simulink model "Example_InterpretedFunction"  (R2024a)
settings: Solver=VariableStepAuto  StartTime=0.0  StopTime=10.0  RelTol=1e-3
values from neighbouring files (symbols this model uses):
  x = acosd(y)    [MATLAB_Cheat_Sheet_Practice.m]
  y = pi    (= 3.14159265359)    [MATLAB_Cheat_Sheet_Practice.m]
undefined symbols (not defined in the file or in its folder): Hello___Matlab
settings Model: Creator=AbdelrahmanMourad  LastModifiedBy=AbdelrahmanMourad

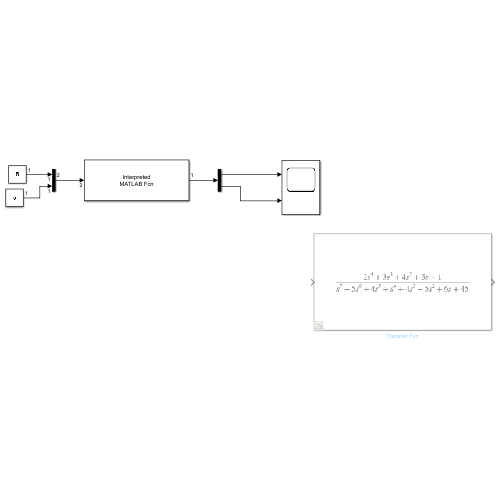
[thumbnail: Simulink's stored preview of the top-level diagram]
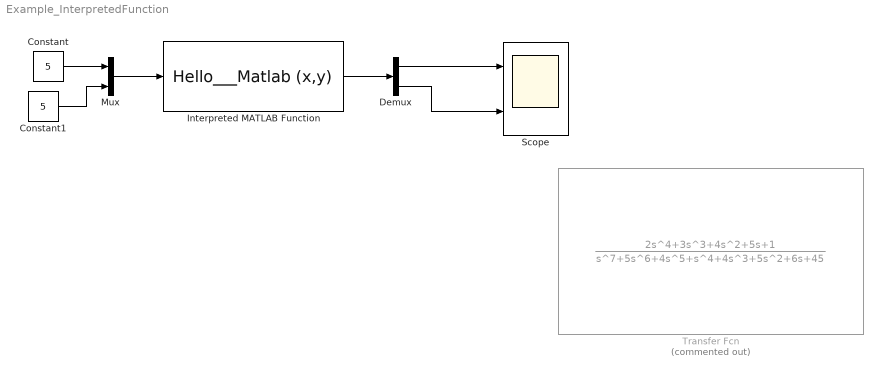
== system Example_InterpretedFunction ==
  Constant : Constant  Value=5  OutDataTypeStr=double
  Constant1 : Constant  Value=5  OutDataTypeStr=double
  Demux : Demux  Outputs=2
  Interpreted MATLAB Function : MATLABFcn  MATLABFcn=Hello___Matlab (x,y)
  Mux : Mux  Inputs=2
  Scope : Scope  NumInputPorts=2
  Transfer Fcn : TransferFcn  Commented=on  Numerator=[2 3 4 5 1]  Denominator=[1 5 4 1 4 5 6 45 ]
  wires:
  Constant/1 -> Mux/1
  Constant1/1 -> Mux/2
  Mux/1 -> Interpreted MATLAB Function/1
  Interpreted MATLAB Function/1 -> Demux/1
  Demux/1 -> Scope/1
  Demux/2 -> Scope/2
